simulink model "mainV02_26"  (R2016b)
settings: Solver=VariableStepAuto  StartTime=0.0  StopTime=Inf  FixedStep=0.001  MaxStep=0.2  RelTol=1e-2
undefined symbols (not defined in the file): checks, deltae_degrees, deltafl_degrees, deltafr_degrees, deltar_degrees, deltat_1, deltat_2, deltat_3, deltat_4, deltat_5, Earth, F, ft, groundReaction, initialValues, LD, Light, m, MIL, Newton, Raphson, s, sigbuilder_block, WGS84
libraries: aerolibutil x19, simulink x10, aerolibtransform2 x6, aerolibasang x4, aerolib6dofsys x4, aerolib6dof2 x4, aerolibwind2 x3, aerolibbdyn x3, aerolibconvert2 x3, aerolibconvert x2, vrlib x2, aerolibatmos2 x1
(part 1 of 5)
settings Model: Creator=Uxío  LastModifiedBy=sork9
settings DataIOCC: ReturnWorkspaceOutputs=on  ReturnWorkspaceOutputsName=spidata
settings OptimizationCC: EfficientMapNaN2IntZero=off  SimCompilerOptimization=on
settings DebuggingCC: ReadBeforeWriteMsg=DisableAll  WriteAfterWriteMsg=DisableAll  WriteAfterReadMsg=DisableAll  MultiTaskDSMMsg=none
settings HardwareCC: TargetBitPerPointer=64  TargetBitPerSizeT=64  TargetBitPerPtrDiffT=64  TargetLongLongMode=on  TargetIntDivRoundTo=Zero  TargetEndianess=LittleEndian  TargetWordSize=64  TargetHWDeviceType=MATLAB Host  ProdEqTarget=off
settings ModelReferenceCC: UpdateModelReferenceTargets=IfOutOfDate
settings SFSimCC: SFSimEcho=off
settings CodeAppCC: MaxIdLength=128
settings GRTTargetCC: TargetLangStandard=C89/C90 (ANSI)  CombineOutputUpdateFcns=off  GRTInterface=on
settings ConfigComp: PSAutoStubLUT=on

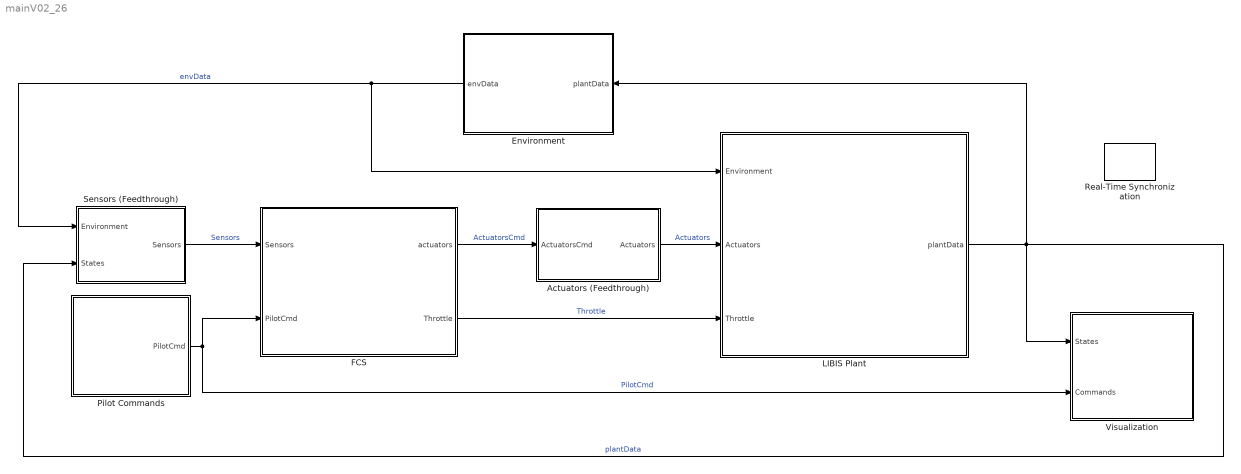
== system mainV02_26 ==
  Actuators (Feedthrough) : Subsystem
  Environment : Subsystem
      mask Display:
      | imageName='Wind.png';
      | currentPath=get_param(bdroot, 'FileName');
      | positions=strfind(currentPath,'\');
      | imagePath=strcat(currentPath(1:positions(end-1)),'graphics\',imageName);
      | image(imagePath);
  FCS : Subsystem
      mask Display:
      | imageName='FCS.png';
      | currentPath=get_param(bdroot, 'FileName');
      | positions=strfind(currentPath,'\');
      | imagePath=strcat(currentPath(1:positions(end-1)),'graphics\',imageName);
      | image(imagePath);
  LIBIS Plant : Subsystem
      mask Display:
      | imageName='LIBIS_Plant.jpg';
      | currentPath=get_param(bdroot, 'FileName');
      | positions=strfind(currentPath,'\');
      | imagePath=strcat(currentPath(1:positions(end-1)),'graphics\',imageName);
      | image(imagePath);
  Pilot Commands : Subsystem  VariantControl=Variants.Command==0
      mask Display:
      | imageName='Pilot.png';
      | currentPath=get_param(bdroot, 'FileName');
      | positions=strfind(currentPath,'\');
      | imagePath=strcat(currentPath(1:positions(end-1)),'graphics\',imageName);
      | image(imagePath);
  Real-Time Synchronization : sldrtlib/Real-Time Synchronization  SampleTime=0.1  MaxMissedTicks=25  ShowMissedTicks=off  YieldWhenWaiting=off
  Sensors (Feedthrough) : Subsystem
  Visualization : Subsystem
  wires:
  FCS/2(Throttle) -> LIBIS Plant/3(Throttle)  "Throttle"
  LIBIS Plant/1(plantData) -> Sensors (Feedthrough)/2(States), Visualization/1(States), Environment/1(plantData)  "plantData"
  Pilot Commands/1(PilotCmd) -> FCS/2(PilotCmd), Visualization/2(Commands)  "PilotCmd"
  Sensors (Feedthrough)/1(Sensors) -> FCS/1(Sensors)  "Sensors"
  Environment/1(envData) -> Sensors (Feedthrough)/1(Environment), LIBIS Plant/1(Environment)  "envData"
  FCS/1(actuators) -> Actuators (Feedthrough)/1(ActuatorsCmd)  "ActuatorsCmd"
  Actuators (Feedthrough)/1(Actuators) -> LIBIS Plant/2(Actuators)  "Actuators"

== system mainV02_26/Actuators (Feedthrough) ==
  ActuatorsCmd : Inport
  Actuators : Outport
  wires:
  ActuatorsCmd/1 -> Actuators/1

== system mainV02_26/Environment ==
  plantData : Inport  OutDataTypeStr=Bus: plantDataBus
  Bus Selector : BusSelector  OutputSignals=LLA.Altitude_m,X_ned,V_ned,Omega_body,CG,DCM_body_earth,LLA.Latitude_deg
  COESA Atmosphere Model : aerolibatmos2/COESA Atmosphere Model  units=Metric (MKS)  spec=1976 COESA-extended U.S. Standard Atmosphere  model=Profile  profile_var=High temperature  profile_percent=1%  profile_alt=5 km (16404 ft)  envelope_var=High temperature  envelope_percent=1%  action=None
  Gravity in Earth Axes : Gain  Gain=[0 0 LD.Inertia.mass]  SaturateOnIntegerOverflow=on  OutDataTypeStr=Inherit: Same as input  ParamDataTypeStr=Inherit: Same as input
  IC : InitialCondition  Value=[0 0 0]
  Math Function : Math  Operator=transpose  SaturateOnIntegerOverflow=on
  Reshape : Reshape
  Reshape1 : Reshape
  Reshape2 : Reshape
  Terrain : Subsystem
  To Body Axes : Product  Multiplication=Matrix(*)  SaturateOnIntegerOverflow=on  InputSameDT=on  OutDataTypeStr=Inherit: Same as first input
  WGS84 Gravity Model : aerolibobsolete/WGS84 Gravity Model  model=WGS84 Taylor Series  units=Metric (MKS)  no_atmos=on  precessing=on  month=February  day=1  year=2000  no_centrifugal=on  action=None
  Wind Models : Subsystem
  envDataBus : BusCreator  Inputs='h_ground','Fground','Mground','windVelocity','windOmega','T','a','P','AirDensity','Fgravity'  OutDataTypeStr=Bus: envDataBus  NonVirtualBus=on
  envData : Outport  OutDataTypeStr=Bus: envDataBus  InitialOutput=0
  wires:
  [Altitude] -> COESA Atmosphere Model/1
  Bus Selector/6 -> To Body Axes/1, Wind Models/3(DCM_be), Terrain/4(DCM_body_earth)  "<DCM_body_earth>"
  Bus Selector/7 -> WGS84 Gravity Model/2  "<Latitude_deg>"
  Bus Selector/3 -> Terrain/2(Ve), Wind Models/1(Ve)  "<V_ned>"
  [Altitude] -> WGS84 Gravity Model/1
  envDataBus/1 -> envData/1  "envData"
  To Body Axes/1 -> Reshape/1  "Fg"
  Wind Models/2(windOmega) -> envDataBus/5  "windOmega"
  Bus Selector/2 -> Terrain/1(Xe)  "<X_ned>"
  WGS84 Gravity Model/1 -> Gravity in Earth Axes/1
  COESA Atmosphere Model/3 -> envDataBus/8  "P"
  COESA Atmosphere Model/2 -> envDataBus/7  "a"
  Wind Models/1(windVelocity) -> envDataBus/4  "windVelocity"
  [Altitude] -> Wind Models/2(Altitude)
  COESA Atmosphere Model/1 -> envDataBus/6  "T"
  COESA Atmosphere Model/4 -> envDataBus/9  "AirDensity"
  Terrain/1(hground) -> envDataBus/1  "h_ground"
  Bus Selector/1 -> [Altitude]  "<Altitude_m>"
  Gravity in Earth Axes/1 -> Math Function/1
  Math Function/1 -> To Body Axes/2
  Reshape/1 -> envDataBus/10  "Fgravity"
  Reshape1/1 -> envDataBus/2  "Fground"
  plantData/1 -> Bus Selector/1
  Bus Selector/5 -> Terrain/5("CG ")  "<CG>"
  Reshape2/1 -> envDataBus/3  "Mground"
  Bus Selector/4 -> Terrain/3("Omega_body ")  "<Omega_body>"
  Terrain/2(Fground) -> IC/1
  Terrain/3(Mground) -> Reshape2/1
  IC/1 -> Reshape1/1

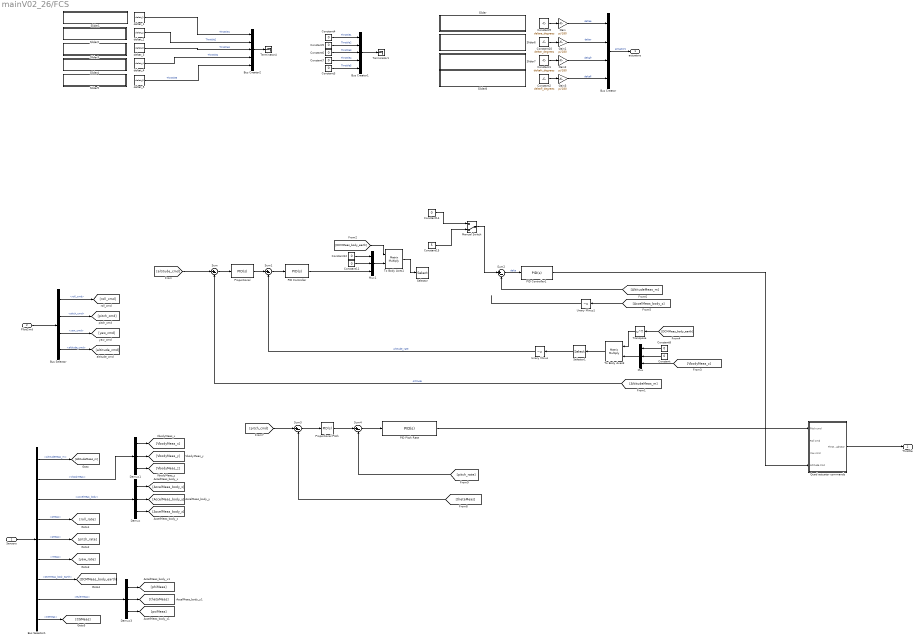
== system mainV02_26/FCS ==
  Sensors : Inport  OutDataTypeStr=Bus: SensorsBus
  PilotCmd : Inport  Port=2  OutDataTypeStr=Bus: CommandBus
  Bus Creator : BusCreator  Inputs=4
  Bus Creator1 : BusCreator  Inputs=5
  Bus Creator2 : BusCreator  Inputs=5
  Bus Selector : BusSelector  OutputSignals=roll_cmd,pitch_cmd,yaw_cmd,altitude_cmd
  Bus Selector1 : BusSelector  OutputSignals=LLAMeas.AltitudeMeas_m,VbodyMeas,AccelMeas_body,OmegaMeas_body.pMeas,OmegaMeas_body.qMeas,OmegaMeas_body.rMeas,DCMMeas_body_earth,EulerMeas,CGMeas
  Constant{,3..8,11..12,14} (10 alike) : Constant  Value=0
  Constant1 : Constant  Value=deltafr_degrees
  Constant10 : Constant  Value=deltar_degrees
  Constant15 : Constant  Value=5
  Constant2 : Constant  Value=deltafl_degrees
  Constant9 : Constant  Value=deltae_degrees
  Demux : Demux  Outputs=3
  Demux1 : Demux  Outputs=3
  Demux3 : Demux  Outputs=3
  Gain{,1..3} (4 alike) : Gain  Gain=pi/180
  Manual Switch : ManualSwitch  CurrentSetting=0
  Mux : Mux  Inputs=3
  Mux1 : Mux  Inputs=3
  PID Controller : simulink/Continuous/PID Controller  Controller=PID  TimeDomain=Continuous-time  SampleTime=-1  IntegratorMethod=Forward Euler  FilterMethod=Forward Euler  Form=Parallel  UseFilter=on  ControllerParametersSource=internal  P=1  I=1  D=0  N=100  InitialConditionSource=internal  InitialConditionForIntegrator=0  InitialConditionForFilter=0  ExternalReset=none  LimitOutput=on  UpperSaturationLimit=1.5*9.81  LowerSaturationLimit=0.5*9.81  LinearizeAsGain=on  AntiWindupMode=none  Kb=1  TrackingMode=off  Kt=1  PParamMin=[]  PParamMax=[]  IParamMin=[]  IParamMax=[]  DParamMin=[]  DParamMax=[]  NParamMin=[]  NParamMax=[]  KbParamMin=[]  KbParamMax=[]  KtParamMin=[]  KtParamMax=[]  POutMin=[]  POutMax=[]  IOutMin=[]  IOutMax=[]  DOutMin=[]  DOutMax=[]  NOutMin=[]  NOutMax=[]  KbOutMin=[]  KbOutMax=[]  KtOutMin=[]  KtOutMax=[]  IntegratorOutMin=[]  IntegratorOutMax=[]  FilterOutMin=[]  FilterOutMax=[]  SumOutMin=[]  SumOutMax=[]  SumI1OutMin=[]  SumI1OutMax=[]  SumI2OutMin=[]  SumI2OutMax=[]  SumI3OutMin=[]  SumI3OutMax=[]  SumDOutMin=[]  SumDOutMax=[]  SaturationOutMin=[]  SaturationOutMax=[]  IntegratorContinuousStateAttributes=''  IntegratorStateMustResolveToSignalObject=off  IntegratorRTWStateStorageClass=Auto  FilterContinuousStateAttributes=''  FilterStateMustResolveToSignalObject=off  FilterRTWStateStorageClass=Auto  DifferentiatorICPrevScaledInput=0  DifferentiatorOutMin=[]  DifferentiatorOutMax=[]
  PID Controller1 : simulink/Continuous/PID Controller  Controller=PID  TimeDomain=Continuous-time  SampleTime=-1  IntegratorMethod=Forward Euler  FilterMethod=Forward Euler  Form=Parallel  UseFilter=on  ControllerParametersSource=internal  P=0.5  I=0.25  D=0.5  N=100  InitialConditionSource=internal  InitialConditionForIntegrator=0  InitialConditionForFilter=0  ExternalReset=none  LimitOutput=on  UpperSaturationLimit=1  LowerSaturationLimit=0  LinearizeAsGain=on  AntiWindupMode=clamping  Kb=1  TrackingMode=off  Kt=1  PParamMin=[]  PParamMax=[]  IParamMin=[]  IParamMax=[]  DParamMin=[]  DParamMax=[]  NParamMin=[]  NParamMax=[]  KbParamMin=[]  KbParamMax=[]  KtParamMin=[]  KtParamMax=[]  POutMin=[]  POutMax=[]  IOutMin=[]  IOutMax=[]  DOutMin=[]  DOutMax=[]  NOutMin=[]  NOutMax=[]  KbOutMin=[]  KbOutMax=[]  KtOutMin=[]  KtOutMax=[]  IntegratorOutMin=[]  IntegratorOutMax=[]  FilterOutMin=[]  FilterOutMax=[]  SumOutMin=[]  SumOutMax=[]  SumI1OutMin=[]  SumI1OutMax=[]  SumI2OutMin=[]  SumI2OutMax=[]  SumI3OutMin=[]  SumI3OutMax=[]  SumDOutMin=[]  SumDOutMax=[]  SaturationOutMin=[]  SaturationOutMax=[]  IntegratorContinuousStateAttributes=''  IntegratorStateMustResolveToSignalObject=off  IntegratorRTWStateStorageClass=Auto  FilterContinuousStateAttributes=''  FilterStateMustResolveToSignalObject=off  FilterRTWStateStorageClass=Auto  DifferentiatorICPrevScaledInput=0  DifferentiatorOutMin=[]  DifferentiatorOutMax=[]
  PID Pitch Rate : simulink/Continuous/PID Controller  Controller=PID  TimeDomain=Continuous-time  SampleTime=-1  IntegratorMethod=Forward Euler  FilterMethod=Forward Euler  Form=Parallel  UseFilter=on  ControllerParametersSource=internal  P=2  I=0  D=0  N=100  InitialConditionSource=internal  InitialConditionForIntegrator=0  InitialConditionForFilter=0  ExternalReset=none  LimitOutput=on  UpperSaturationLimit=1  LowerSaturationLimit=0  LinearizeAsGain=on  AntiWindupMode=none  Kb=1  TrackingMode=off  Kt=1  PParamMin=[]  PParamMax=[]  IParamMin=[]  IParamMax=[]  DParamMin=[]  DParamMax=[]  NParamMin=[]  NParamMax=[]  KbParamMin=[]  KbParamMax=[]  KtParamMin=[]  KtParamMax=[]  POutMin=[]  POutMax=[]  IOutMin=[]  IOutMax=[]  DOutMin=[]  DOutMax=[]  NOutMin=[]  NOutMax=[]  KbOutMin=[]  KbOutMax=[]  KtOutMin=[]  KtOutMax=[]  IntegratorOutMin=[]  IntegratorOutMax=[]  FilterOutMin=[]  FilterOutMax=[]  SumOutMin=[]  SumOutMax=[]  SumI1OutMin=[]  SumI1OutMax=[]  SumI2OutMin=[]  SumI2OutMax=[]  SumI3OutMin=[]  SumI3OutMax=[]  SumDOutMin=[]  SumDOutMax=[]  SaturationOutMin=[]  SaturationOutMax=[]  IntegratorContinuousStateAttributes=''  IntegratorStateMustResolveToSignalObject=off  IntegratorRTWStateStorageClass=Auto  FilterContinuousStateAttributes=''  FilterStateMustResolveToSignalObject=off  FilterRTWStateStorageClass=Auto  DifferentiatorICPrevScaledInput=0  DifferentiatorOutMin=[]  DifferentiatorOutMax=[]
  Proportional : simulink/Continuous/PID Controller  Controller=PID  TimeDomain=Continuous-time  SampleTime=-1  IntegratorMethod=Forward Euler  FilterMethod=Forward Euler  Form=Parallel  UseFilter=on  ControllerParametersSource=internal  P=-1  I=0  D=0  N=100  InitialConditionSource=internal  InitialConditionForIntegrator=0  InitialConditionForFilter=0  ExternalReset=none  LimitOutput=on  UpperSaturationLimit=250  LowerSaturationLimit=-inf  LinearizeAsGain=on  AntiWindupMode=none  Kb=1  TrackingMode=off  Kt=1  PParamMin=[]  PParamMax=[]  IParamMin=[]  IParamMax=[]  DParamMin=[]  DParamMax=[]  NParamMin=[]  NParamMax=[]  KbParamMin=[]  KbParamMax=[]  KtParamMin=[]  KtParamMax=[]  POutMin=[]  POutMax=[]  IOutMin=[]  IOutMax=[]  DOutMin=[]  DOutMax=[]  NOutMin=[]  NOutMax=[]  KbOutMin=[]  KbOutMax=[]  KtOutMin=[]  KtOutMax=[]  IntegratorOutMin=[]  IntegratorOutMax=[]  FilterOutMin=[]  FilterOutMax=[]  SumOutMin=[]  SumOutMax=[]  SumI1OutMin=[]  SumI1OutMax=[]  SumI2OutMin=[]  SumI2OutMax=[]  SumI3OutMin=[]  SumI3OutMax=[]  SumDOutMin=[]  SumDOutMax=[]  SaturationOutMin=[]  SaturationOutMax=[]  IntegratorContinuousStateAttributes=''  IntegratorStateMustResolveToSignalObject=off  IntegratorRTWStateStorageClass=Auto  FilterContinuousStateAttributes=''  FilterStateMustResolveToSignalObject=off  FilterRTWStateStorageClass=Auto  DifferentiatorICPrevScaledInput=0  DifferentiatorOutMin=[]  DifferentiatorOutMax=[]
  Proportional Pitch : simulink/Continuous/PID Controller  Controller=PID  TimeDomain=Continuous-time  SampleTime=-1  IntegratorMethod=Forward Euler  FilterMethod=Forward Euler  Form=Parallel  UseFilter=on  ControllerParametersSource=internal  P=4  I=0  D=0  N=100  InitialConditionSource=internal  InitialConditionForIntegrator=0  InitialConditionForFilter=0  ExternalReset=none  LimitOutput=off  UpperSaturationLimit=inf  LowerSaturationLimit=-inf  LinearizeAsGain=on  AntiWindupMode=none  Kb=1  TrackingMode=off  Kt=1  PParamMin=[]  PParamMax=[]  IParamMin=[]  IParamMax=[]  DParamMin=[]  DParamMax=[]  NParamMin=[]  NParamMax=[]  KbParamMin=[]  KbParamMax=[]  KtParamMin=[]  KtParamMax=[]  POutMin=[]  POutMax=[]  IOutMin=[]  IOutMax=[]  DOutMin=[]  DOutMax=[]  NOutMin=[]  NOutMax=[]  KbOutMin=[]  KbOutMax=[]  KtOutMin=[]  KtOutMax=[]  IntegratorOutMin=[]  IntegratorOutMax=[]  FilterOutMin=[]  FilterOutMax=[]  SumOutMin=[]  SumOutMax=[]  SumI1OutMin=[]  SumI1OutMax=[]  SumI2OutMin=[]  SumI2OutMax=[]  SumI3OutMin=[]  SumI3OutMax=[]  SumDOutMin=[]  SumDOutMax=[]  SaturationOutMin=[]  SaturationOutMax=[]  IntegratorContinuousStateAttributes=''  IntegratorStateMustResolveToSignalObject=off  IntegratorRTWStateStorageClass=Auto  FilterContinuousStateAttributes=''  FilterStateMustResolveToSignalObject=off  FilterRTWStateStorageClass=Auto  DifferentiatorICPrevScaledInput=0  DifferentiatorOutMin=[]  DifferentiatorOutMax=[]
  Quad actuator commands : Subsystem
  Selector : Selector  InputPortWidth=3  IndexOptions=Index vector (dialog)  Indices=[ 3]  OutputSizes=1
  Selector1 : Selector  InputPortWidth=3  IndexOptions=Index vector (dialog)  Indices=[ 3]  OutputSizes=1
  Slider : Subsystem  DialogController=hmiCreateDDGDialog  IsWebBlock=on  mask(MWDashboardBlock){webBlockId=6273dd38-214f-4c77-9b1a-24b6ec7057c4, webBlockType=slider, ShowInLibBrowser=on, ShowInitialText=on, HMISrcModelName=mainV02_26}
      mask prompts: webBlockId "WebBlock Id"; webBlockType "WebBlock Type"; HMISrcModelName "Source Model"
      mask help: SimulinkHMI:dialogs:SliderDialogDesc
      mask Help: helpview([docroot '/mapfiles/simulink.map'], 'hmi_slider')
      mask Display:
      | if strcmp(get_param(bdroot(gcb),'BlockDiagramType'), 'library')
      |     image([(matlabroot) '/toolbox/simulink/hmi/icons/Slider.png']);
      | end
  Slider1 : Subsystem  DialogController=hmiCreateDDGDialog  IsWebBlock=on  mask(MWDashboardBlock){webBlockId=70020a0d-53bd-4fc8-9fe2-57375c6f10bc, webBlockType=slider, ShowInLibBrowser=on, ShowInitialText=on, HMISrcModelName=mainV02_26}
      mask prompts: webBlockId "WebBlock Id"; webBlockType "WebBlock Type"; HMISrcModelName "Source Model"
      mask help: SimulinkHMI:dialogs:SliderDialogDesc
      mask Help: helpview([docroot '/mapfiles/simulink.map'], 'hmi_slider')
      mask Display:
      | if strcmp(get_param(bdroot(gcb),'BlockDiagramType'), 'library')
      |     image([(matlabroot) '/toolbox/simulink/hmi/icons/Slider.png']);
      | end
  Slider2 : Subsystem  DialogController=hmiCreateDDGDialog  IsWebBlock=on  mask(MWDashboardBlock){webBlockId=1c2f52ab-856d-4c73-8b77-5cca8dc888a8, webBlockType=slider, ShowInLibBrowser=on, ShowInitialText=on, HMISrcModelName=mainV02_26}
      mask prompts: webBlockId "WebBlock Id"; webBlockType "WebBlock Type"; HMISrcModelName "Source Model"
      mask help: SimulinkHMI:dialogs:SliderDialogDesc
      mask Help: helpview([docroot '/mapfiles/simulink.map'], 'hmi_slider')
      mask Display:
      | if strcmp(get_param(bdroot(gcb),'BlockDiagramType'), 'library')
      |     image([(matlabroot) '/toolbox/simulink/hmi/icons/Slider.png']);
      | end
  Slider3 : Subsystem  DialogController=hmiCreateDDGDialog  IsWebBlock=on  mask(MWDashboardBlock){webBlockId=06ca73c2-e5c3-419a-af4c-8301bb851811, webBlockType=slider, ShowInLibBrowser=on, ShowInitialText=on, HMISrcModelName=mainV02_26}
      mask prompts: webBlockId "WebBlock Id"; webBlockType "WebBlock Type"; HMISrcModelName "Source Model"
      mask help: SimulinkHMI:dialogs:SliderDialogDesc
      mask Help: helpview([docroot '/mapfiles/simulink.map'], 'hmi_slider')
      mask Display:
      | if strcmp(get_param(bdroot(gcb),'BlockDiagramType'), 'library')
      |     image([(matlabroot) '/toolbox/simulink/hmi/icons/Slider.png']);
      | end
  Slider4 : Subsystem  DialogController=hmiCreateDDGDialog  IsWebBlock=on  mask(MWDashboardBlock){webBlockId=0f1aa799-7d0b-4e65-9c98-585766d84b05, webBlockType=slider, ShowInLibBrowser=on, ShowInitialText=on, HMISrcModelName=mainV02_26}
      mask prompts: webBlockId "WebBlock Id"; webBlockType "WebBlock Type"; HMISrcModelName "Source Model"
      mask help: SimulinkHMI:dialogs:SliderDialogDesc
      mask Help: helpview([docroot '/mapfiles/simulink.map'], 'hmi_slider')
      mask Display:
      | if strcmp(get_param(bdroot(gcb),'BlockDiagramType'), 'library')
      |     image([(matlabroot) '/toolbox/simulink/hmi/icons/Slider.png']);
      | end
  Slider5 : Subsystem  DialogController=hmiCreateDDGDialog  IsWebBlock=on  mask(MWDashboardBlock){webBlockId=1aba3140-aa7a-42dc-9545-4aab801dd215, webBlockType=slider, ShowInLibBrowser=on, ShowInitialText=on, HMISrcModelName=mainV02_26}
      mask prompts: webBlockId "WebBlock Id"; webBlockType "WebBlock Type"; HMISrcModelName "Source Model"
      mask help: SimulinkHMI:dialogs:SliderDialogDesc
      mask Help: helpview([docroot '/mapfiles/simulink.map'], 'hmi_slider')
      mask Display:
      | if strcmp(get_param(bdroot(gcb),'BlockDiagramType'), 'library')
      |     image([(matlabroot) '/toolbox/simulink/hmi/icons/Slider.png']);
      | end
  Slider6 : Subsystem  DialogController=hmiCreateDDGDialog  IsWebBlock=on  mask(MWDashboardBlock){webBlockId=3d9f47b7-f15d-42be-b3f0-4bf7c2d4a508, webBlockType=slider, ShowInLibBrowser=on, ShowInitialText=on, HMISrcModelName=mainV02_26}
      mask prompts: webBlockId "WebBlock Id"; webBlockType "WebBlock Type"; HMISrcModelName "Source Model"
      mask help: SimulinkHMI:dialogs:SliderDialogDesc
      mask Help: helpview([docroot '/mapfiles/simulink.map'], 'hmi_slider')
      mask Display:
      | if strcmp(get_param(bdroot(gcb),'BlockDiagramType'), 'library')
      |     image([(matlabroot) '/toolbox/simulink/hmi/icons/Slider.png']);
      | end
  Slider7 : Subsystem  DialogController=hmiCreateDDGDialog  IsWebBlock=on  mask(MWDashboardBlock){webBlockId=8e5c7658-11f4-4f70-8154-234cc52576e8, webBlockType=slider, ShowInLibBrowser=on, ShowInitialText=on, HMISrcModelName=mainV02_26}
      mask prompts: webBlockId "WebBlock Id"; webBlockType "WebBlock Type"; HMISrcModelName "Source Model"
      mask help: SimulinkHMI:dialogs:SliderDialogDesc
      mask Help: helpview([docroot '/mapfiles/simulink.map'], 'hmi_slider')
      mask Display:
      | if strcmp(get_param(bdroot(gcb),'BlockDiagramType'), 'library')
      |     image([(matlabroot) '/toolbox/simulink/hmi/icons/Slider.png']);
      | end
  Slider8 : Subsystem  DialogController=hmiCreateDDGDialog  IsWebBlock=on  mask(MWDashboardBlock){webBlockId=fd4f6454-3dcd-4a0d-9f3e-71aa520b8d15, webBlockType=slider, ShowInLibBrowser=on, ShowInitialText=on, HMISrcModelName=mainV02_26}
      mask prompts: webBlockId "WebBlock Id"; webBlockType "WebBlock Type"; HMISrcModelName "Source Model"
      mask help: SimulinkHMI:dialogs:SliderDialogDesc
      mask Help: helpview([docroot '/mapfiles/simulink.map'], 'hmi_slider')
      mask Display:
      | if strcmp(get_param(bdroot(gcb),'BlockDiagramType'), 'library')
      |     image([(matlabroot) '/toolbox/simulink/hmi/icons/Slider.png']);
      | end
  Sum{,1..4} (5 alike) : Sum  Inputs=|+-
  Terminator1 : Terminator
  Terminator4 : Terminator
  To Body Axes1 : Product  Multiplication=Matrix(*)  SaturateOnIntegerOverflow=on  InputSameDT=on  OutDataTypeStr=Inherit: Same as first input
  To Body Axes3 : Product  Multiplication=Matrix(*)  SaturateOnIntegerOverflow=on  InputSameDT=on  OutDataTypeStr=Inherit: Same as first input
  Transpose : Math  Operator=transpose  SaturateOnIntegerOverflow=on
  Unary Minus : UnaryMinus
  Unary Minus1 : UnaryMinus
  deltat_1 : Constant  Value=deltat_1
  deltat_2 : Constant  Value=deltat_2
  deltat_3 : Constant  Value=deltat_3
  deltat_4 : Constant  Value=deltat_4
  deltat_5 : Constant  Value=deltat_5
  actuators : Outport
  Throttle : Outport  Port=2
  wires:
  PilotCmd/1 -> Bus Selector/1
  Sensors/1 -> Bus Selector1/1
  Bus Creator/1 -> actuators/1  "actuators"
  Gain1/1 -> Bus Creator/2  "deltar"
  Gain2/1 -> Bus Creator/3  "deltafr"
  Gain3/1 -> Bus Creator/4  "deltafl"
  Constant4/1 -> Bus Creator1/1  "Throttle1"
  Constant6/1 -> Bus Creator1/3  "Throttle3"
  Constant5/1 -> Bus Creator1/2  "Throttle2"
  Gain/1 -> Bus Creator/1  "deltae"
  deltat_1/1 -> Bus Creator2/1  "Throttle1"
  deltat_3/1 -> Bus Creator2/3  "Throttle3"
  deltat_2/1 -> Bus Creator2/2  "Throttle2"
  deltat_4/1 -> Bus Creator2/4  "Throttle4"
  deltat_5/1 -> Bus Creator2/5  "Throttle5"
  Constant10/1 -> Gain1/1
  Constant1/1 -> Gain2/1
  Constant2/1 -> Gain3/1
  Constant7/1 -> Bus Creator1/4  "Throttle4"
  Constant3/1 -> Bus Creator1/5  "Throttle5"
  Bus Selector1/1 -> [AltitudeMeas_m]  "<AltitudeMeas_m>"
  Bus Creator2/1 -> Terminator4/1
  Bus Selector/1 -> [roll_cmd]  "<roll_cmd>"
  Bus Selector/2 -> [pitch_cmd]  "<pitch_cmd>"
  Bus Selector/3 -> [yaw_cmd]  "<yaw_cmd>"
  Bus Selector/4 -> [altitude_cmd]  "<altitude_cmd>"
  Bus Selector1/4 -> [roll_rate]  "<pMeas>"
  Bus Selector1/5 -> [pitch_rate]  "<qMeas>"
  Bus Selector1/6 -> [yaw_rate]  "<rMeas>"
  Bus Selector1/3 -> Demux/1  "<AccelMeas_body>"
  Demux/1 -> [AccelMeas_body_x]
  Demux/2 -> [AccelMeas_body_y]
  Demux/3 -> [AccelMeas_body_z]
  [altitude_cmd] -> Sum/1
  [AltitudeMeas_m] -> Sum/2  "Altitude"
  Sum/1 -> Proportional/1
  Proportional/1 -> Sum1/1
  Sum1/1 -> PID Controller/1
  Constant8/1 -> Mux/1
  Constant/1 -> Mux/2
  Mux/1 -> To Body Axes3/2
  Constant11/1 -> Mux1/2
  Constant12/1 -> Mux1/1
  Mux1/1 -> To Body Axes1/2
  PID Controller/1 -> Mux1/3
  [DCMMeas_body_earth] -> To Body Axes1/1
  To Body Axes1/1 -> Selector/1
  Bus Selector1/7 -> [DCMMeas_body_earth]  "<DCMMeas_body_earth>"
  Demux1/1 -> [VbodyMeas_x]
  Demux1/2 -> [VbodyMeas_y]
  Demux1/3 -> [VbodyMeas_z]
  Bus Selector1/2 -> Demux1/1  "<VbodyMeas>"
  [VbodyMeas_z] -> Mux/3
  [DCMMeas_body_earth] -> Transpose/1
  Transpose/1 -> To Body Axes3/1
  To Body Axes3/1 -> Selector1/1
  Selector1/1 -> Unary Minus/1
  Sum2/1 -> PID Controller1/1  "delta"
  [AccelMeas_body_z] -> Unary Minus1/1
  PID Controller1/1 -> Quad actuator commands/4(Altitude cmd)
  Unary Minus/1 -> Sum1/2  "Altitude_rate"
  Constant14/1 -> Manual Switch/1
  Manual Switch/1 -> Sum2/1
  Constant15/1 -> Manual Switch/2
  Unary Minus1/1 -> ?
  [AltitudeMeas_m] -> Sum2/2
  Bus Selector1/8 -> Demux3/1  "<EulerMeas>"
  Demux3/1 -> [phiMeas]
  Demux3/2 -> [thetaMeas]
  Demux3/3 -> [psiMeas]
  [thetaMeas] -> Sum3/2
  Sum3/1 -> Proportional Pitch/1
  [pitch_rate] -> Sum4/2
  Proportional Pitch/1 -> Sum4/1
  Sum4/1 -> PID Pitch Rate/1
  PID Pitch Rate/1 -> Quad actuator commands/1(Pitch cmd)
  Constant9/1 -> Gain/1
  [pitch_cmd] -> Sum3/1
  Bus Creator1/1 -> Terminator1/1
  Bus Selector1/9 -> [CGMeas]  "<CGMeas>"
  Quad actuator commands/1(Throttle_Quadrotor) -> Throttle/1

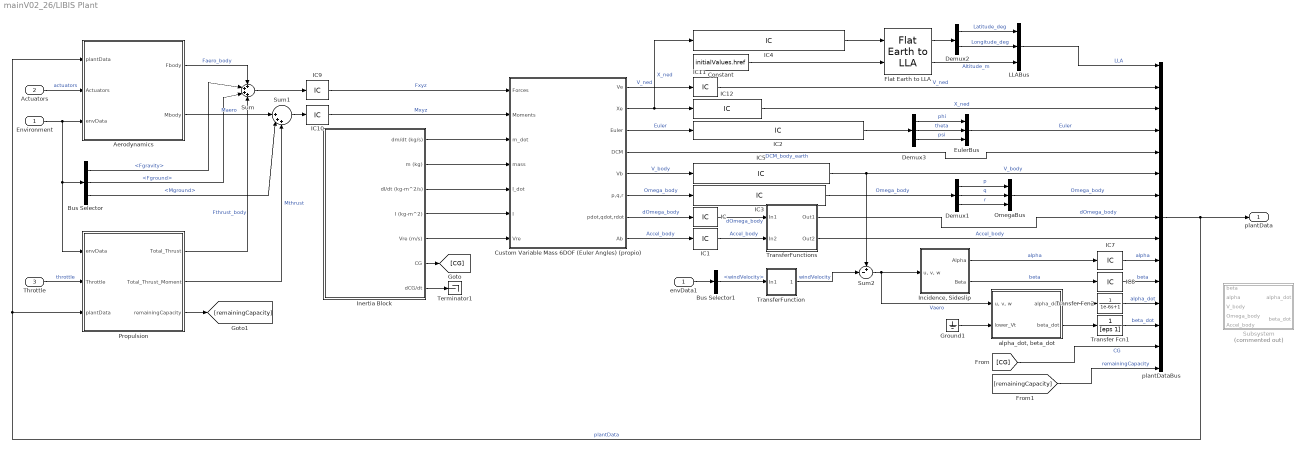
== system mainV02_26/LIBIS Plant ==
  Environment : Inport  OutDataTypeStr=Bus: envDataBus
  Actuators : Inport  Port=2
  Throttle : Inport  Port=3
  Aerodynamics : Subsystem
  Bus Selector : BusSelector  OutputSignals=Fgravity,Fground,Mground
  Bus Selector1 : BusSelector  OutputSignals=windVelocity
  Constant : Constant  Value=initialValues.href
  Custom Variable Mass 6DOF (Euler Angles) (propio) : Subsystem  mask(6DOF EoM (Body Axis)){units=Metric (MKS), mtype=Custom Variable, rep=Euler Angles, xme_0=[initialValues.Xe0 initialValues.Ye0 initialValues.Ze0], Vm_0=[initialValues.u0 initialValues.v0 initialValues.w0], eul_0=[initialValues.roll0 initialValues.pitch0 initialValues.yaw0], pm_0=[initialValues.p0 initialValues.q0 initialValues.r0], mass_0=1.0, mass_e=0.5, mass_f=2.0, inertia=eye(3), inertia_e=eye(3), inertia_f=2*eye(3), k_quat=1.0, vre_flag=on}
      mask prompts: units "aeroblks:aeroblk6dofbody:block6DOFEoMBodyAxisParamUnits"; mtype "aeroblks:aeroblk6dofbody:block6DOFEoMBodyAxisParamMasstype"; rep "aeroblks:aeroblk6dofbody:block6DOFEoMBodyAxisParamRepresentation"; xme_0 "aeroblks:aeroblk6dofbody:block6DOFEoMBodyAxisParamInitialpositionininertialaxesXeYeZe"; Vm_0 "aeroblks:aeroblk6dofbody:block6DOFEoMBodyAxisParamInitialvelocityinbodyaxesUvw"; eul_0 "aeroblks:aeroblk6dofbody:block6DOFEoMBodyAxisParamInitialEulerorientationrollpitchyaw"; pm_0 "aeroblks:aeroblk6dofbody:block6DOFEoMBodyAxisParamInitialbodyrotationratespqr"; mass_0 "aeroblks:aeroblk6dofbody:block6DOFEoMBodyAxisParamInitialmass"; mass_e "aeroblks:aeroblk6dofbody:block6DOFEoMBodyAxisParamEmptymass"; mass_f "aeroblks:aeroblk6dofbody:block6DOFEoMBodyAxisParamFullmass"; inertia "aeroblks:aeroblk6dofbody:block6DOFEoMBodyAxisParamInertia"; inertia_e "aeroblks:aeroblk6dofbody:block6DOFEoMBodyAxisParamEmptyinertiamatrix"; inertia_f "aeroblks:aeroblk6dofbody:block6DOFEoMBodyAxisParamFullinertiamatrix"; k_quat "aeroblks:aeroblk6dofbody:block6DOFEoMBodyAxisParamGainforquaternionnormalization"; vre_flag "aeroblks:aeroblk6dofbody:block6DOFEoMBodyAxisParamIncludemassflowrelativevelocity"
      mask help: aeroblks:aeroblk6dofbody:block6DOFEoMBodyAxisDesc
      mask init:
      | ports=aeroicon('aeroblk6dofbody','icon');
      mask Help: eval('asbhelp(''custom_variable_mass_sixdof_euler_angles'')');
      mask TypeOptions units: aeroblks:aeroblk6dofbody:block6DOFEoMBodyAxisParamComboMetricMKS | aeroblks:aeroblk6dofbody:block6DOFEoMBodyAxisParamComboEnglishVelocityinfts | aeroblks:aeroblk6dofbody:block6DOFEoMBodyAxisParamComboEnglishVelocityinkts
      mask TypeOptions mtype: aeroblks:aeroblk6dofbody:block6DOFEoMBodyAxisParamComboFixed | aeroblks:aeroblk6dofbody:block6DOFEoMBodyAxisParamComboSimpleVariable | aeroblks:aeroblk6dofbody:block6DOFEoMBodyAxisParamComboCustomVariable
      mask Callback mtype: aeroicon('aeroblk6dofbody');
      mask TypeOptions rep: aeroblks:aeroblk6dofbody:block6DOFEoMBodyAxisParamComboEulerAngles | aeroblks:aeroblk6dofbody:block6DOFEoMBodyAxisParamComboQuaternion
      mask Callback rep: aeroicon('aeroblk6dofbody');
      mask Display:
      | port_label(ports(1).type,ports(1).port,ports(1).txt,'texmode','on');
      | port_label(ports(2).type,ports(2).port,ports(2).txt,'texmode','on');
      | port_label(ports(3).type,ports(3).port,ports(3).txt,'texmode','on');
      | port_label(ports(4).type,ports(4).port,ports(4).txt,'texmode','on');
      | port_label(ports(5).type,ports(5).port,ports(5).txt,'texmode','on');
      | port_label(ports(6).type,ports(6).port,ports(6).txt,'texmode','on');
      | port_label(ports(7).type,ports(7).port,ports(7).txt,'texmode','on');
      | port_label(ports(8).type,ports(8).port,ports(8).txt,'texmode','on');
      | port_label(ports(9).type,ports(9).port,ports(9).txt,'texmode','on');
      | port_label(ports(10).type,ports(10).port,ports(10).txt,'texmode','on');
      | port_label(ports(11).type,ports(11).port,ports(11).txt,'texmode','on');
      | port_label(ports(12).type,ports(12).port,ports(12).txt,'texmode','on');
      | port_label(ports(13).type,ports(13).port,ports(13).txt,'texmode','on');
      | port_label(ports(14).type,ports(14).port,ports(14).txt,'texmode','on');
      | port_label(ports(15).type,ports(15).port,ports(15).txt,'texmode','on');
      | port_label(ports(16).type,ports(16).port,ports(16).txt,'texmode','on');
      | [x y xp yp highstr lowstr maxy miny]=aeroimage('sixdofbody',gcbh);
      | text(0.5,maxy+0.065,highstr{:},'horizontalAlignment','center')
      | text(0.5,miny-0.06,lowstr{:},'horizontalAlignment','center')
      | plot(x,y);
      | patch(xp, yp);
  Demux1 : Demux  Outputs=3
  Demux2 : Demux  Outputs=2
  Demux3 : Demux  Outputs=3
  EulerBus : BusCreator  Inputs='phi','theta','psi'  OutDataTypeStr=Bus: EulerBus  NonVirtualBus=on
  Flat Earth to LLA : aerolibtransform2/Flat Earth to LLA  units=Metric (MKS)  ptype=Earth (WGS84)  F=1/298.257223563  R=6378137  LL0=initialValues.LatLong0  psi=initialValues.heading0
  Ground1 : Ground
  IC{,1,9..11} (5 alike) : InitialCondition  Value=[0 0 0]
  IC12 : InitialCondition  Value=[0 0 -initialValues.href]
  IC2 : InitialCondition  Value=[initialValues.roll0, initialValues.pitch0, initialValues.yaw0]
  IC3 : InitialCondition  Value=[initialValues.p0 initialValues.q0 initialValues.r0]
  IC4 : InitialCondition  Value=[initialValues.Xe0 initialValues.Ye0 initialValues.Ze0]
  IC5 : InitialCondition  Value=[initialValues.u0 initialValues.v0 initialValues.w0]
  IC7 : InitialCondition  Value=0
  IC8 : InitialCondition  Value=0
  "Incidence, Sideslip" : Subsystem
  Inertia Block : Subsystem
      mask Display:
      | imageName='Moment_of_inertia.png';
      | currentPath=get_param(bdroot, 'FileName');
      | positions=strfind(currentPath,'\');
      | imagePath=strcat(currentPath(1:positions(end-1)),'graphics\',imageName);
      | image(imagePath);
  LLABus : BusCreator  Inputs='Latitude_deg','Longitude_deg','Altitude_m'  OutDataTypeStr=Bus: LLABus  NonVirtualBus=on
  OmegaBus : BusCreator  Inputs='p','q','r'  OutDataTypeStr=Bus: OmegaBus  NonVirtualBus=on
  Propulsion : Subsystem
  Subsystem : Subsystem  Commented=on
  Sum : Sum  Inputs=++++
  Sum1 : Sum  Inputs=||+++
  Sum2 : Sum  Inputs=+-|
  Terminator1 : Terminator
  Transfer Fcn1 : TransferFcn  Denominator=[eps 1]
  Transfer Fcn2 : TransferFcn  Denominator=[1e-6 1]
  TransferFunction : Subsystem
  TransferFunctions : Subsystem
  "alpha_dot, beta_dot" : Subsystem
  envData1 : InportShadow  OutDataTypeStr=Bus: envDataBus
  plantDataBus : BusCreator  Inputs='LLA','V_ned','X_ned','Euler','DCM_body_earth','V_body','Omega_body','dOmega_body','Accel_body','alpha','beta','alpha_dot','beta_dot','CG','remainingCapacity'  OutDataTypeStr=Bus: plantDataBus  NonVirtualBus=on
  plantData : Outport  OutDataTypeStr=Bus: plantDataBus
  wires:
  Inertia Block/4(I (kg-m^2)) -> Custom Variable Mass 6DOF (Euler Angles) (propio)/6(I)
  plantDataBus/1 -> Aerodynamics/1(plantData), Propulsion/3(plantData), plantData/1  "plantData"
  Flat Earth to LLA/2 -> LLABus/3  "Altitude_m"
  Custom Variable Mass 6DOF (Euler Angles) (propio)/2(Xe) -> IC12/1, IC4/1  "X_ned"
  Custom Variable Mass 6DOF (Euler Angles) (propio)/3(Euler) -> IC2/1  "Euler"
  EulerBus/1 -> plantDataBus/4  "Euler"
  Flat Earth to LLA/1 -> Demux2/1
  Demux2/1 -> LLABus/1  "Latitude_deg"
  Inertia Block/2(m (kg)) -> Custom Variable Mass 6DOF (Euler Angles) (propio)/4(mass)
  Inertia Block/5(Vre (m/s)) -> Custom Variable Mass 6DOF (Euler Angles) (propio)/7(Vre)
  Custom Variable Mass 6DOF (Euler Angles) (propio)/5(Vb) -> IC5/1  "V_body"
  Inertia Block/7(dCG/dt) -> Terminator1/1
  [CG] -> plantDataBus/14  "CG"
  Custom Variable Mass 6DOF (Euler Angles) (propio)/4(DCM) -> plantDataBus/5  "DCM_body_earth"
  Inertia Block/3(dI/dt (kg-m^2/s)) -> Custom Variable Mass 6DOF (Euler Angles) (propio)/5(I_dot)
  LLABus/1 -> plantDataBus/1  "LLA"
  "Incidence, Sideslip"/1(Alpha) -> IC7/1  "alpha"
  Demux3/1 -> EulerBus/1  "phi"
  Demux3/3 -> EulerBus/3  "psi"
  Inertia Block/6(CG) -> [CG]
  Inertia Block/1(dm/dt (kg/s)) -> Custom Variable Mass 6DOF (Euler Angles) (propio)/3(m_dot)
  Constant/1 -> Flat Earth to LLA/2
  Demux2/2 -> LLABus/2  "Longitude_deg"
  "Incidence, Sideslip"/2(Beta) -> IC8/1  "beta"
  Demux3/2 -> EulerBus/2  "theta"
  Custom Variable Mass 6DOF (Euler Angles) (propio)/1(Ve) -> IC11/1  "V_ned"
  OmegaBus/1 -> plantDataBus/7  "Omega_body"
  Custom Variable Mass 6DOF (Euler Angles) (propio)/6(p,q,r) -> IC3/1  "Omega_body"
  Demux1/2 -> OmegaBus/2  "q"
  Demux1/1 -> OmegaBus/1  "p"
  Demux1/3 -> OmegaBus/3  "r"
  Actuators/1 -> Aerodynamics/2(Actuators)  "actuators"
  Throttle/1 -> Propulsion/2(Throttle)  "throttle"
  Propulsion/3(remainingCapacity) -> [remainingCapacity]
  [remainingCapacity] -> plantDataBus/15  "remainingCapacity"
  Propulsion/1(Total_Thrust) -> Sum/4  "Fthrust_body"
  Environment/1 -> Propulsion/1(envData), Bus Selector/1, Aerodynamics/3(envData)
  IC4/1 -> Flat Earth to LLA/1
  IC5/1 -> plantDataBus/6, Sum2/1  "V_body"
  IC3/1 -> Demux1/1  "Omega_body"
  IC2/1 -> Demux3/1
  Bus Selector/1 -> Sum/2  "<Fgravity>"
  IC7/1 -> plantDataBus/10  "alpha"
  envData1/1 -> Bus Selector1/1
  Bus Selector/2 -> Sum/3  "<Fground>"
  Bus Selector1/1 -> TransferFunction/1(In1)  "<windVelocity>"
  Sum2/1 -> "alpha_dot, beta_dot"/1("u, v, w"), "Incidence, Sideslip"/1("u, v, w")  "Vaero"
  Custom Variable Mass 6DOF (Euler Angles) (propio)/7(pdot,qdot,rdot) -> IC/1  "dOmega_body"
  Custom Variable Mass 6DOF (Euler Angles) (propio)/8(Ab) -> IC1/1  "Accel_body"
  IC8/1 -> plantDataBus/11  "beta"
  Sum1/1 -> IC10/1
  Sum/1 -> IC9/1
  IC9/1 -> Custom Variable Mass 6DOF (Euler Angles) (propio)/1(Forces)  "Fxyz"
  IC10/1 -> Custom Variable Mass 6DOF (Euler Angles) (propio)/2(Moments)  "Mxyz"
  IC/1 -> TransferFunctions/1(In1)  "dOmega_body"
  IC1/1 -> TransferFunctions/2(In2)  "Accel_body"
  TransferFunctions/1(Out1) -> plantDataBus/8  "dOmega_body"
  TransferFunctions/2(Out2) -> plantDataBus/9  "Accel_body"
  IC11/1 -> plantDataBus/2  "V_ned"
  IC12/1 -> plantDataBus/3  "X_ned"
  Transfer Fcn1/1 -> plantDataBus/13  "beta_dot"
  TransferFunction/1(Out1) -> Sum2/2  "windVelocity"
  Transfer Fcn2/1 -> plantDataBus/12  "alpha_dot"
  Aerodynamics/2(Mbody) -> Sum1/1  "Maero"
  Aerodynamics/1(Fbody) -> Sum/1  "Faero_body"
  "alpha_dot, beta_dot"/1(alpha_dot) -> Transfer Fcn2/1
  "alpha_dot, beta_dot"/2(beta_dot) -> Transfer Fcn1/1
  Ground1/1 -> "alpha_dot, beta_dot"/2(lower_Vt)
  Bus Selector/3 -> Sum1/2  "<Mground>"
  Propulsion/2(Total_Thrust_Moment) -> Sum1/3  "Mthrust"

== system mainV02_26/Pilot Commands ==
  Bus Creator : BusCreator  Inputs=9  OutDataTypeStr=Bus: CommandBus  NonVirtualBus=on
  Signal Builder : Subsystem  Tag=STV Subsys  LoadFcn=sigbuilder_block('load');  StartFcn=sigbuilder_block('start');  StopFcn=sigbuilder_block('stop');  ClipboardFcn=sigbuilder_block('clipboard');  mask(Sigbuilder block){tuvar=[0:10]}
      mask help: Simulink:masks:SigbuilderBlock_MD
      mask init:
      | if ~strcmp(get_param(bdroot(gcbh),'SimulationStatus'),'stopped') tuvar = sigbuilder_block('maskInit'); end
      settings: CopyFcn=sigbuilder_block('copy');  DeleteFcn=sigbuilder_block('delete');  ModelCloseFcn=sigbuilder_block('modelClose');  PreSaveFcn=sigbuilder_block('preSave');  PauseFcn=sigbuilder_block('pause');  ContinueFcn=sigbuilder_block('continue');  NameChangeFcn=sigbuilder_block('namechange');  OpenFcn=sigbuilder_block('open',[234 6 960 605.25 ]);  CloseFcn=sigbuilder_block('close');
      mask Display: plot(0, 0, 100, 100,[2, 2, 32, 32, 2], [68, 8, 8, 68, 68],[32, 2], [38, 38], [32, 19, 2],[53, 60, 44], [32, 17, 17, 2],[16, 16, 31, 31]);txt = getActiveGroup(gcbh);text(2, 100, txt,'verticalAlignment', 'top');
  PilotCmd : Outport  OutDataTypeStr=Bus: CommandBus
  wires:
  Bus Creator/1 -> PilotCmd/1
  Signal Builder/1(Roll) -> Bus Creator/1  "roll_cmd"
  Signal Builder/2(Pitch) -> Bus Creator/2  "pitch_cmd"
  Signal Builder/3(Yaw) -> Bus Creator/3  "yaw_cmd"
  Signal Builder/4(Altitude) -> Bus Creator/4  "altitude_cmd"
  Signal Builder/9(Throttle5) -> Bus Creator/9  "Throttle5_cmd"
  Signal Builder/8(Throttle4) -> Bus Creator/8  "Throttle4_cmd"
  Signal Builder/7(Throttle3) -> Bus Creator/7  "Throttle3_cmd"
  Signal Builder/6(Throttle2) -> Bus Creator/6  "Throttle2_cmd"
  Signal Builder/5(Throttle1) -> Bus Creator/5  "Throttle1_cmd"

== system mainV02_26/Sensors (Feedthrough) ==
  Environment : Inport  OutDataTypeStr=Bus: envDataBus
  States : Inport  Port=2  OutDataTypeStr=Bus: plantDataBus
  Bus Creator2 : BusCreator  Inputs='LLAMeas','VbodyMeas','AccelMeas_body','OmegaMeas_body','DCMMeas_body_earth','EulerMeas','VaeroMeas_body','alphaMeas','betaMeas','CGMeas','remainingCapacityMeas'  OutDataTypeStr=Bus: SensorsBus  NonVirtualBus=on
  CPU : Subsystem
  GPS : Subsystem
  IMU : Subsystem
  Pitot : Subsystem
  Veleta : Subsystem
  Sensors : Outport  OutDataTypeStr=Bus: SensorsBus
  wires:
  Environment/1 -> IMU/2(Environment), Pitot/1(Environment)
  GPS/1(LLAMeas) -> Bus Creator2/1  "LLAMeas"
  Bus Creator2/1 -> Sensors/1  "Sensors"
  States/1 -> GPS/1(States), IMU/1(States), Pitot/2(States), CPU/1(States), Veleta/1(States)
  IMU/1(VbodyMeas) -> Bus Creator2/2  "VbodyMeas"
  IMU/2(AccelMeas_body) -> Bus Creator2/3  "AccelMeas_body"
  IMU/3(OmegaMeas_body) -> Bus Creator2/4  "OmegaMeas_body"
  IMU/4(DCMMeas_body_earth) -> Bus Creator2/5  "DCMMeas_body_earth"
  IMU/5(EulerMeas) -> Bus Creator2/6  "EulerMeas"
  Pitot/1(VaeroMeas_body) -> Bus Creator2/7  "VaeroMeas_body"
  Veleta/1(alphaMeas) -> Bus Creator2/8  "alphaMeas"
  Veleta/2(betaMeas) -> Bus Creator2/9  "betaMeas"
  CPU/2(remainingCapacityMeas) -> Bus Creator2/11  "remainingCapacityMeas"
  CPU/1(CGMeas) -> Bus Creator2/10  "CGMeas"

== system mainV02_26/Visualization ==
  States : Inport  OutDataTypeStr=Bus: plantDataBus
  Commands : Inport  Port=2  OutDataTypeStr=Bus: CommandBus
  Airspeed Indicator : Subsystem  DialogController=aeroblksHMICreateDDGDialog  IsWebBlock=on  mask(MWDashboardBlock){webBlockId=1660c180-4922-4edc-b12a-b6c4fb3472e7, webBlockType=airspeedindicator, ShowInLibBrowser=on, ShowInitialText=on, HMISrcModelName=mainV02_26}
      mask prompts: webBlockId "WebBlock Id"; webBlockType "WebBlock Type"; HMISrcModelName "Source Model"
      mask help: aeroblksHMI:aeroblkhmi:AirspeedIndicatorDialogDesc
      mask Help: eval('asbhmihelp(''airspeedindicator'')');
      mask Display:
      | if strcmp(get_param(bdroot(gcb),'BlockDiagramType'), 'library')
      |  image([(matlabroot) '/toolbox/aeroblks/aeroblks/hmi/icons/AirspeedIndicatorIcon.svg'])
      | end
  Alpha and beta visualization : Scope  NumInputPorts=2
  Altimeter : Subsystem  DialogController=aeroblksHMICreateDDGDialog  IsWebBlock=on  mask(MWDashboardBlock){webBlockId=dac4b64b-8b08-4b88-951c-85bcef5f9a8d, webBlockType=altimeter, ShowInLibBrowser=on, ShowInitialText=on, HMISrcModelName=mainV02_26}
      mask prompts: webBlockId "WebBlock Id"; webBlockType "WebBlock Type"; HMISrcModelName "Source Model"
      mask help: aeroblksHMI:aeroblkhmi:AltimeterDialogDesc
      mask Help: eval('asbhmihelp(''altimeter'')');
      mask Display:
      | if strcmp(get_param(bdroot(gcb),'BlockDiagramType'), 'library')
      |  image([(matlabroot) '/toolbox/aeroblks/aeroblks/hmi/icons/AltimeterIcon.svg'])
      | end
  Altitude : Scope
  Artificial Horizon : Subsystem  DialogController=aeroblksHMICreateDDGDialog  IsWebBlock=on  mask(MWDashboardBlock){webBlockId=71b89583-386f-4e5a-a87e-fbc6faf0c9b0, webBlockType=artificialhorizon, ShowInLibBrowser=on, ShowInitialText=on, HMISrcModelName=mainV02_26}
      mask prompts: webBlockId "WebBlock Id"; webBlockType "WebBlock Type"; HMISrcModelName "Source Model"
      mask help: aeroblksHMI:aeroblkhmi:ArtificialHorizonDialogDesc
      mask Help: eval('asbhmihelp(''artificialhorizon'')');
      mask Display:
      | if strcmp(get_param(bdroot(gcb),'BlockDiagramType'), 'library')
      |  image([(matlabroot) '/toolbox/aeroblks/aeroblks/hmi/icons/ArtificialHorizonIcon.svg'])
      | end
  Axes to VR Axes : Subsystem
  Bus Selector : BusSelector  OutputSignals=X_ned
  Bus Selector1 : BusSelector  OutputSignals=Euler.phi,Euler.theta,Euler.psi
  Bus Selector2 : BusSelector  OutputSignals=LLA.Altitude_m
  Bus Selector3 : BusSelector  OutputSignals=V_body,V_ned
  Bus Selector4 : BusSelector  OutputSignals=alpha,beta
  Climb Rate Indicator : Subsystem  DialogController=aeroblksHMICreateDDGDialog  IsWebBlock=on  mask(MWDashboardBlock){webBlockId=2290786a-142e-4cdc-9e89-cbe88d1b2ef4, webBlockType=climbindicator, ShowInLibBrowser=on, ShowInitialText=on, HMISrcModelName=mainV02_26}
      mask prompts: webBlockId "WebBlock Id"; webBlockType "WebBlock Type"; HMISrcModelName "Source Model"
      mask help: aeroblksHMI:aeroblkhmi:ClimbIndicatorDialogDesc
      mask Help: eval('asbhmihelp(''climbindicator'')');
      mask Display:
      | if strcmp(get_param(bdroot(gcb),'BlockDiagramType'), 'library')
      |  image([(matlabroot) '/toolbox/aeroblks/aeroblks/hmi/icons/ClimbIndicatorIcon.svg'])
      | end
  Demux : Demux  Outputs=3
  Demux1 : Demux  Outputs=3
  Demux2 : Demux  Outputs=3
  Earth position : Scope  NumInputPorts=3
  Euler angles visualization : Scope  NumInputPorts=3
  Euler to VR : Subsystem
  Heading Indicator : Subsystem  DialogController=aeroblksHMICreateDDGDialog  IsWebBlock=on  mask(MWDashboardBlock){webBlockId=f0aafb45-9505-4aed-89ac-b6a93bae7c37, webBlockType=headingindicator, ShowInLibBrowser=on, ShowInitialText=on, HMISrcModelName=mainV02_26}
      mask prompts: webBlockId "WebBlock Id"; webBlockType "WebBlock Type"; HMISrcModelName "Source Model"
      mask help: aeroblksHMI:aeroblkhmi:HeadingIndicatorDialogDesc
      mask Help: eval('asbhmihelp(''headingindicator'')');
      mask Display:
      | if strcmp(get_param(bdroot(gcb),'BlockDiagramType'), 'library')
      |  image([(matlabroot) '/toolbox/aeroblks/aeroblks/hmi/icons/HeadingIndicatorIcon.svg'])
      | end
  Mux : Mux  Inputs=3
  Rate Transition : RateTransition
  Rate Transition1 : RateTransition
  Subsystem : Subsystem
  Terminator{,1..5} (6 alike) : Terminator
  VR Sink : vrlib/VR Sink  InstantiateOnLoad=on  SampleTime=0.1  ViewEnable=on  RemoteChange=off  RemoteView=off  FieldsWritten=HL20.rotation.4.1.1.double#HL20.translation.3.1.1.double  WorldFileName=aeroblk_HL20.wrl  WorldDescription=aeroblk_HL20  AutoView=off  VideoDimensions=[]  AllowVariableSize=off
  VR Sink1 : vrlib/VR Sink  InstantiateOnLoad=on  SampleTime=0.1  ViewEnable=on  RemoteChange=off  RemoteView=off  FieldsWritten=Plane.rotation.4.1.1.double#Plane.translation.3.1.1.double  WorldFileName=.\graphics\vr01.wrl  WorldDescription=VR Plane Take-Off  AutoView=on  VideoDimensions=[]  AllowVariableSize=off  mask(Virtual Reality Sink){}
      mask Display:
      | % This is a new mask on top of the base mask.
      | % Use "View base mask" link below to see the base mask.
      | imageName='vr01.wrl.thumbnail.png';
      | currentPath=get_param(bdroot, 'FileName');
      | positions=strfind(currentPath,'\');
      | imagePath=strcat(currentPath(1:positions(end-1)),'graphics\',imageName);
      | image(imagePath);
  V_body visualization : Scope  NumInputPorts=3
  V_ned visualization : Scope  NumInputPorts=3
  wires:
  Bus Selector1/1 -> Euler angles visualization/1, Mux/1  "<phi>"
  Bus Selector1/2 -> Mux/2, Euler angles visualization/2  "<theta>"
  Bus Selector1/3 -> Euler angles visualization/3, Mux/3  "<psi>"
  States/1 -> Bus Selector/1, Bus Selector1/1, Bus Selector4/1, Bus Selector3/1, Bus Selector2/1
  Bus Selector2/1 -> Altitude/1  "<Altitude_m>"
  Euler to VR/1(Axis Angle) -> Rate Transition/1
  Axes to VR Axes/1(Xe VR) -> Rate Transition1/1
  Bus Selector/1 -> Demux/1, Axes to VR Axes/1(Xe), Subsystem/1("X_ned ")  "<X_ned>"
  Mux/1 -> Subsystem/2(Euler_angles), Euler to VR/1(Euler Angles)
  Bus Selector3/1 -> Demux2/1, Subsystem/3(V_body)  "<V_body>"
  Bus Selector3/2 -> Demux1/1, Subsystem/4(V_ned)  "<V_ned>"
  Subsystem/1(Airspeed (kts)) -> Terminator/1
  Subsystem/2(Height (ft)) -> Terminator1/1
  Subsystem/3(Roll Flightpath (deg)) -> Terminator2/1
  Subsystem/4(Climb Rate (ft/min)) -> Terminator3/1
  Subsystem/5(Heading (deg)) -> Terminator4/1
  Demux/2 -> Earth position/2
  Demux/1 -> Earth position/1
  Demux/3 -> Earth position/3
  Bus Selector4/1 -> Alpha and beta visualization/1  "<alpha>"
  Bus Selector4/2 -> Alpha and beta visualization/2  "<beta>"
  Demux1/1 -> V_ned visualization/1  "V_ned_x"
  Demux1/2 -> V_ned visualization/2  "V_ned_y"
  Demux1/3 -> V_ned visualization/3  "V_ned_z"
  Demux2/1 -> V_body visualization/1  "V_body_x"
  Demux2/2 -> V_body visualization/2  "V_body_y"
  Demux2/3 -> V_body visualization/3  "V_body_z"
  Rate Transition/1 -> VR Sink1/1, VR Sink/1  "rotation"
  Rate Transition1/1 -> VR Sink1/2, VR Sink/2  "translation"
  Commands/1 -> Terminator5/1

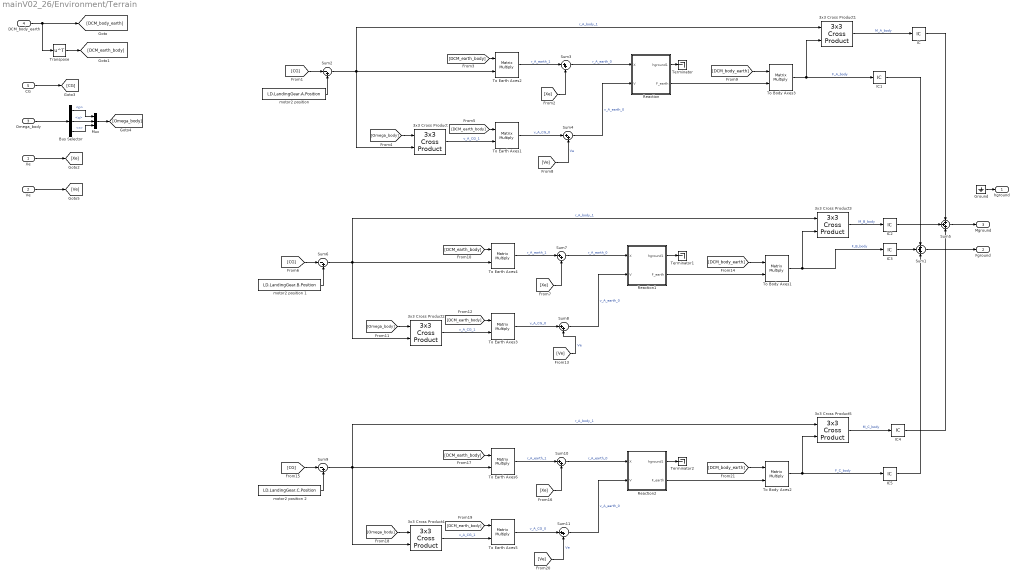
== system mainV02_26/Environment/Terrain ==
  Xe : Inport  Unit=m
  Ve : Inport  Port=2
  "Omega_body " : Inport  Port=3
  DCM_body_earth : Inport  Port=4
  "CG " : Inport  Port=5
  3x3 Cross Product{,1..5} (6 alike) : aerolibutil/3x3 Cross Product
  Bus Selector : BusSelector  OutputSignals=p,q,r
  Ground : Ground
  IC{,1..5} (6 alike) : InitialCondition  Value=[0 0 0]
  Mux : Mux  Inputs=3
  Reaction : Subsystem
  Reaction1 : Subsystem
  Reaction2 : Subsystem
  Sum1 : Sum  Inputs=+++
  Sum{3..4,7..8,10..11} (6 alike) : Sum  Inputs=|++
  Sum2 : Sum  Inputs=|-+
  Sum5 : Sum  Inputs=+++
  Sum6 : Sum  Inputs=|-+
  Sum9 : Sum  Inputs=|-+
  Terminator : Terminator
  Terminator1 : Terminator
  Terminator2 : Terminator
  To Body Axes1 : Product  Multiplication=Matrix(*)  SaturateOnIntegerOverflow=on  InputSameDT=on  OutDataTypeStr=Inherit: Same as first input
  To Body Axes2 : Product  Multiplication=Matrix(*)  SaturateOnIntegerOverflow=on  InputSameDT=on  OutDataTypeStr=Inherit: Same as first input
  To Body Axes3 : Product  Multiplication=Matrix(*)  SaturateOnIntegerOverflow=on  InputSameDT=on  OutDataTypeStr=Inherit: Same as first input
  To Earth Axes{1..6} (6 alike) : Product  Multiplication=Matrix(*)  SaturateOnIntegerOverflow=on  InputSameDT=on  OutDataTypeStr=Inherit: Same as first input
  Transpose : Math  Operator=transpose  SaturateOnIntegerOverflow=on
  "motor2 position " : Constant  Value=LD.LandingGear.A.Position
  motor2 position 1 : Constant  Value=LD.LandingGear.B.Position
  motor2 position 2 : Constant  Value=LD.LandingGear.C.Position
  hground : Outport
  Fground : Outport  Port=2
  Mground : Outport  Port=3
  wires:
  DCM_body_earth/1 -> Transpose/1, [DCM_body_earth]
  [DCM_earth_body] -> To Earth Axes2/1
  To Earth Axes2/1 -> Sum3/1  "r_A_earth_1"
  Transpose/1 -> [DCM_earth_body]
  [Xe] -> Sum3/2
  "CG "/1 -> [CG]
  [CG] -> Sum2/1
  "motor2 position "/1 -> Sum2/2
  Sum3/1 -> Reaction/1(X)  "r_A_earth_0"
  Reaction/2(F_earth) -> To Body Axes3/2
  [Omega_body] -> 3x3 Cross Product/1
  3x3 Cross Product/1 -> To Earth Axes1/2  "v_A_CG_1"
  [DCM_earth_body] -> To Earth Axes1/1
  To Earth Axes1/1 -> Sum4/1  "v_A_CG_0"
  Xe/1 -> [Xe]
  Ve/1 -> [Ve]
  [Ve] -> Sum4/2  "Ve"
  Sum4/1 -> Reaction/2(V)  "v_A_earth_0"
  Sum2/1 -> 3x3 Cross Product1/1, To Earth Axes2/2, 3x3 Cross Product/2  "r_A_body_1"
  [DCM_body_earth] -> To Body Axes3/1
  To Body Axes3/1 -> IC1/1, 3x3 Cross Product1/2  "F_A_body"
  3x3 Cross Product1/1 -> IC/1  "M_A_body"
  Sum5/1 -> Mground/1
  Sum1/1 -> Fground/1
  "Omega_body "/1 -> Bus Selector/1
  Bus Selector/1 -> Mux/1  "<p>"
  Bus Selector/2 -> Mux/2  "<q>"
  Bus Selector/3 -> Mux/3  "<r>"
  Mux/1 -> [Omega_body]
  [DCM_earth_body] -> To Earth Axes4/1
  To Earth Axes4/1 -> Sum7/1  "r_A_earth_1"
  [Xe] -> Sum7/2
  [CG] -> Sum6/1
  motor2 position 1/1 -> Sum6/2
  Sum7/1 -> Reaction1/1(X)  "r_A_earth_0"
  Reaction1/2(F_earth) -> To Body Axes1/2
  [Omega_body] -> 3x3 Cross Product2/1
  3x3 Cross Product2/1 -> To Earth Axes3/2  "v_A_CG_1"
  [DCM_earth_body] -> To Earth Axes3/1
  To Earth Axes3/1 -> Sum8/1  "v_A_CG_0"
  [Ve] -> Sum8/2  "Ve"
  Sum8/1 -> Reaction1/2(V)  "v_A_earth_0"
  Sum6/1 -> 3x3 Cross Product3/1, To Earth Axes4/2, 3x3 Cross Product2/2  "r_A_body_1"
  [DCM_body_earth] -> To Body Axes1/1
  To Body Axes1/1 -> 3x3 Cross Product3/2, IC3/1  "F_B_body"
  3x3 Cross Product3/1 -> IC2/1  "M_B_body"
  [DCM_earth_body] -> To Earth Axes6/1
  To Earth Axes6/1 -> Sum10/1  "r_A_earth_1"
  [Xe] -> Sum10/2
  [CG] -> Sum9/1
  motor2 position 2/1 -> Sum9/2
  Sum10/1 -> Reaction2/1(X)  "r_A_earth_0"
  Reaction2/2(F_earth) -> To Body Axes2/2
  [Omega_body] -> 3x3 Cross Product4/1
  3x3 Cross Product4/1 -> To Earth Axes5/2  "v_A_CG_1"
  [DCM_earth_body] -> To Earth Axes5/1
  To Earth Axes5/1 -> Sum11/1  "v_A_CG_0"
  [Ve] -> Sum11/2  "Ve"
  Sum11/1 -> Reaction2/2(V)  "v_A_earth_0"
  Sum9/1 -> 3x3 Cross Product5/1, To Earth Axes6/2, 3x3 Cross Product4/2  "r_A_body_1"
  [DCM_body_earth] -> To Body Axes2/1
  To Body Axes2/1 -> IC5/1, 3x3 Cross Product5/2  "F_C_body"
  3x3 Cross Product5/1 -> IC4/1  "M_C_body"
  IC/1 -> Sum5/1
  IC1/1 -> Sum1/1
  IC2/1 -> Sum5/2
  IC3/1 -> Sum1/2
  IC4/1 -> Sum5/3
  IC5/1 -> Sum1/3
  Ground/1 -> hground/1
  Reaction/1(hground1) -> Terminator/1
  Reaction1/1(hground1) -> Terminator1/1
  Reaction2/1(hground1) -> Terminator2/1
